simulink model "Position_Tilt"  (R2016a)
settings: Solver=ode2  StartTime=0.0  StopTime=10.0  FixedStep=tc  RelTol=1e-3
InitFcn:
  | Parameters
libraries: simulink x2
settings Model: Creator=pela  LastModifiedBy=Claudio
settings DataIOCC: LimitDataPoints=on  SaveFormat=Array
settings HardwareCC: ProdBitPerPointer=32  ProdLargestAtomicInteger=Long  ProdLargestAtomicFloat=Double  ProdIntDivRoundTo=Undefined  ProdWordSize=32  ProdHWDeviceType=ARM Compatible->ARM Cortex
settings ModelReferenceCC: PropagateSignalLabelsOutOfModel=off
settings RTWCC: GenCodeOnly=on  GenerateReport=on  Toolchain=Microsoft Visual C++ 2015 v14.0 | nmake (64-bit Windows)  BuildConfiguration=Faster Runs  LaunchReport=on  TargetLang=C++
settings GRTTargetCC: MatFileLogging=off  MultiInstanceERTCode=on  CodeInterfacePackaging=C++ class  SupportNonFinite=off
settings ConfigComp: CovModelRefEnable=Off

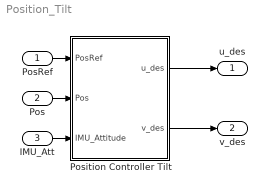
== system Position_Tilt ==
  PosRef : Inport
  Pos : Inport  Port=2
  IMU_Att : Inport  Port=3
  Position Controller Tilt : Subsystem
  u_des : Outport
  v_des : Outport  Port=2
  wires:
  PosRef/1 -> Position Controller Tilt/1(PosRef)
  IMU_Att/1 -> Position Controller Tilt/3(IMU_Attitude)
  Pos/1 -> Position Controller Tilt/2(Pos)
  Position Controller Tilt/2(v_des) -> v_des/1
  Position Controller Tilt/1(u_des) -> u_des/1

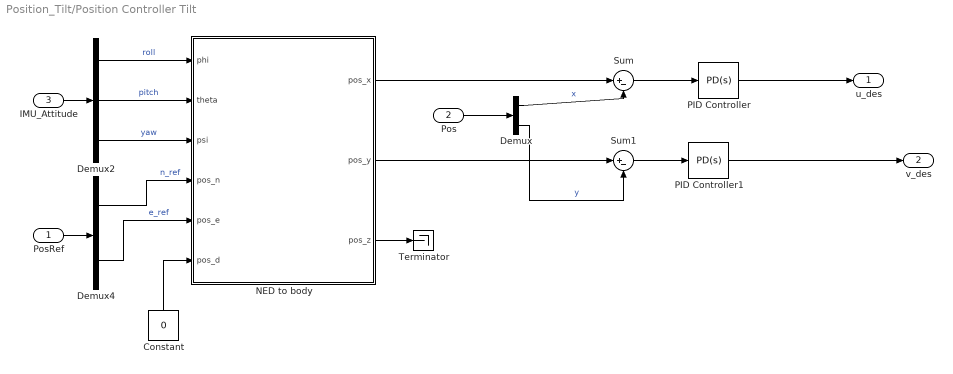
== system Position_Tilt/Position Controller Tilt ==
  PosRef : Inport
  Pos : Inport  Port=2
  IMU_Attitude : Inport  Port=3
  Constant : Constant  Value=0
  Demux : Demux  Outputs=2
  Demux2 : Demux  Outputs=3
  Demux4 : Demux  Outputs=2
  NED to body : MATLAB Function  TreatAsAtomicUnit=on
  PID Controller : simulink/Continuous/PID Controller  Controller=PD  TimeDomain=Continuous-time  SampleTime=-1  IntegratorMethod=Forward Euler  FilterMethod=Forward Euler  Form=Parallel  UseFilter=on  ControllerParametersSource=internal  P=1  I=1  D=0  N=100  InitialConditionSource=internal  InitialConditionForIntegrator=0  InitialConditionForFilter=0  ExternalReset=none  LimitOutput=off  UpperSaturationLimit=inf  LowerSaturationLimit=-inf  LinearizeAsGain=on  AntiWindupMode=none  Kb=1  TrackingMode=off  Kt=1  PParamMin=[]  PParamMax=[]  IParamMin=[]  IParamMax=[]  DParamMin=[]  DParamMax=[]  NParamMin=[]  NParamMax=[]  KbParamMin=[]  KbParamMax=[]  KtParamMin=[]  KtParamMax=[]  POutMin=[]  POutMax=[]  IOutMin=[]  IOutMax=[]  DOutMin=[]  DOutMax=[]  NOutMin=[]  NOutMax=[]  KbOutMin=[]  KbOutMax=[]  KtOutMin=[]  KtOutMax=[]  IntegratorOutMin=[]  IntegratorOutMax=[]  FilterOutMin=[]  FilterOutMax=[]  SumOutMin=[]  SumOutMax=[]  SumI1OutMin=[]  SumI1OutMax=[]  SumI2OutMin=[]  SumI2OutMax=[]  SumI3OutMin=[]  SumI3OutMax=[]  SumDOutMin=[]  SumDOutMax=[]  SaturationOutMin=[]  SaturationOutMax=[]  IntegratorContinuousStateAttributes=''  IntegratorStateMustResolveToSignalObject=off  IntegratorRTWStateStorageClass=Auto  FilterContinuousStateAttributes=''  FilterStateMustResolveToSignalObject=off  FilterRTWStateStorageClass=Auto  DifferentiatorICPrevScaledInput=0  DifferentiatorOutMin=[]  DifferentiatorOutMax=[]
  PID Controller1 : simulink/Continuous/PID Controller  Controller=PD  TimeDomain=Continuous-time  SampleTime=-1  IntegratorMethod=Forward Euler  FilterMethod=Forward Euler  Form=Parallel  UseFilter=on  ControllerParametersSource=internal  P=1  I=1  D=0  N=100  InitialConditionSource=internal  InitialConditionForIntegrator=0  InitialConditionForFilter=0  ExternalReset=none  LimitOutput=off  UpperSaturationLimit=inf  LowerSaturationLimit=-inf  LinearizeAsGain=on  AntiWindupMode=none  Kb=1  TrackingMode=off  Kt=1  PParamMin=[]  PParamMax=[]  IParamMin=[]  IParamMax=[]  DParamMin=[]  DParamMax=[]  NParamMin=[]  NParamMax=[]  KbParamMin=[]  KbParamMax=[]  KtParamMin=[]  KtParamMax=[]  POutMin=[]  POutMax=[]  IOutMin=[]  IOutMax=[]  DOutMin=[]  DOutMax=[]  NOutMin=[]  NOutMax=[]  KbOutMin=[]  KbOutMax=[]  KtOutMin=[]  KtOutMax=[]  IntegratorOutMin=[]  IntegratorOutMax=[]  FilterOutMin=[]  FilterOutMax=[]  SumOutMin=[]  SumOutMax=[]  SumI1OutMin=[]  SumI1OutMax=[]  SumI2OutMin=[]  SumI2OutMax=[]  SumI3OutMin=[]  SumI3OutMax=[]  SumDOutMin=[]  SumDOutMax=[]  SaturationOutMin=[]  SaturationOutMax=[]  IntegratorContinuousStateAttributes=''  IntegratorStateMustResolveToSignalObject=off  IntegratorRTWStateStorageClass=Auto  FilterContinuousStateAttributes=''  FilterStateMustResolveToSignalObject=off  FilterRTWStateStorageClass=Auto  DifferentiatorICPrevScaledInput=0  DifferentiatorOutMin=[]  DifferentiatorOutMax=[]
  Sum : Sum  Inputs=|+-
  Sum1 : Sum  Inputs=|+-
  Terminator : Terminator
  u_des : Outport
  v_des : Outport  Port=2
  wires:
  Demux4/1 -> NED to body/4(pos_n)  "n_ref"
  Demux4/2 -> NED to body/5(pos_e)  "e_ref"
  PosRef/1 -> Demux4/1
  NED to body/3(pos_z) -> Terminator/1
  IMU_Attitude/1 -> Demux2/1
  Demux2/2 -> NED to body/2(theta)  "pitch"
  Constant/1 -> NED to body/6(pos_d)
  Pos/1 -> Demux/1
  Demux2/3 -> NED to body/3(psi)  "yaw"
  Demux2/1 -> NED to body/1(phi)  "roll"
  Sum/1 -> PID Controller/1
  NED to body/1(pos_x) -> Sum/1
  Demux/1 -> Sum/2  "x"
  PID Controller/1 -> u_des/1
  Sum1/1 -> PID Controller1/1
  NED to body/2(pos_y) -> Sum1/1
  Demux/2 -> Sum1/2  "y"
  PID Controller1/1 -> v_des/1

== matlab function Position_Tilt/Position Controller Tilt/NED to body ==
  data: pos_x output; pos_y output; pos_z output; phi input; theta input; psi input; pos_n input; pos_e input; pos_d input
function [pos_x,pos_y,pos_z] = ned2body(phi,theta,psi,pos_n,pos_e,pos_d)
%#codegen
Pos_NED = [pos_n ;
    pos_e ;
    pos_d];

%% Rotate Acc_body to Earth frame
Sphi = sin(phi);
Cphi = cos(phi);
Stheta = sin(theta);
Ctheta = cos(theta);
Spsi = sin(psi);
Cpsi = cos(psi);

Tbe = [           Cpsi*Ctheta,                  Ctheta*Spsi,     -Stheta;
 Cpsi*Sphi*Stheta - Cphi*Spsi, Cphi*Cpsi + Sphi*Spsi*Stheta, Ctheta*Sphi;
 Sphi*Spsi + Cphi*Cpsi*Stheta, Cphi*Spsi*Stheta - Cpsi*Sphi, Cphi*Ctheta];

Tbet = [ Cpsi*Ctheta, Cpsi*Sphi*Stheta - Cphi*Spsi, Sphi*Spsi + Cphi*Cpsi*Stheta ;
         Ctheta*Spsi, Cphi*Cpsi + Sphi*Spsi*Stheta, Cphi*Spsi*Stheta - Cpsi*Sphi ;
             -Stheta,                  Ctheta*Sphi,                  Cphi*Ctheta];

% Acc_Earth = zeros(3,1);

Pos_body = Tbe * Pos_NED ;

pos_x = Pos_body(1);
pos_y = Pos_body(2);
pos_z = Pos_body(3);
